simulink model "hil_demo"  (R2020a)
settings: Solver=VariableStepAuto  StartTime=0.0  StopTime=30  RelTol=1e-3
undefined symbols (not defined in the file): frame, physconst, system, UE
libraries: commsync2 x3, commsink2 x2, commdigbbndpm3 x2, commfilt2 x2, commsequence2 x2, phasedbflib x2, dspmathops x1, phaseddoalib x1, commrfcorlib x1, commutil2 x1, dspstat3 x1, dspsrcs4 x1
settings Model: Creator=jose_  LastModifiedBy=jose_

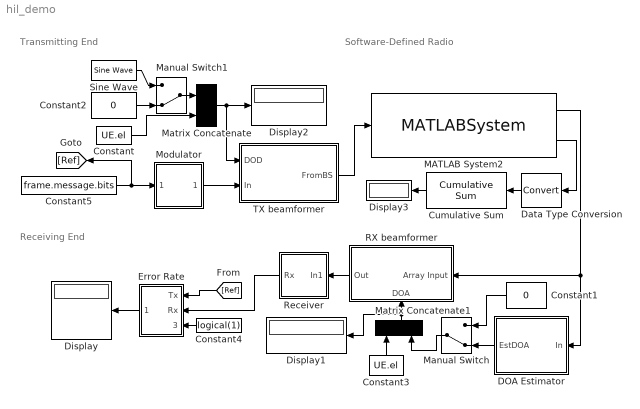
== system hil_demo ==
  note: Receiving End
  note: Software-Defined Radio
  note: Transmitting End
  Constant : Constant  Value=UE.el
  Constant1 : Constant  Value=0
  Constant2 : Constant  Value=0
  Constant3 : Constant  Value=UE.el
  Constant4 : Constant  Value=logical(1)
  Constant5 : Constant  Value=frame.message.bits  SampleTime=system.step
  Cumulative Sum : dspmathops/Cumulative Sum  dim=Channels (running sum)  reset_popup=None  roundingMode=Floor  overflowMode=off  outputDataTypeStr=Inherit: Same as accumulator  outputMin=[]  outputMax=[]  outputLastDataTypeStr=Inherit: Same as accumulator
  DOA Estimator : Subsystem
      mask Display: image('$imagefile'); % Use "Edit Image" on toolstrip to change.
  Data Type Conversion : DataTypeConversion
  Display{,1..3} (4 alike) : Display
  Error Rate : Subsystem
  MATLAB System2 : MATLABSystem  System=bladeRF_MIMO_Simulink  loopback_mode=None  xb200=off  SimulateUsing=Interpreted execution  enable_rx=on  enable_overrun=on  rx_frequency=system.freq  rx_samplerate=SDR.samplerate  rx_bandwidth=1.5  rx_gain=SDR.rx_gain  enable_rx_biastee=off  rx_agc=MANUAL  rx_num_buffers=SDR.stream.n_buffers  rx_num_transfers=SDR.stream.n_transfers  rx_buf_size=SDR.stream.buffer_size  rx_timeout_ms=SDR.stream.timeout  rx_step_size=SDR.samples_per_step  enable_tx=on  enable_underrun=off  tx_frequency=system.freq  tx_samplerate=SDR.samplerate  tx_bandwidth=1.5  tx_gain=SDR.tx_gain  enable_tx_biastee=off  tx_num_buffers=SDR.stream.n_buffers  tx_num_transfers=SDR.stream.n_transfers  tx_buf_size=SDR.stream.buffer_size  tx_timeout_ms=SDR.stream.timeout  tx_step_size=SDR.samples_per_step  verbosity=Verbose
      mask Type: bladeRF_MIMO_Simulink
      mask Display:
      | disp(['Nuand' char(10) 'bladeRF 2.0' char(10) 'MIMO']);
      | port_label('input',1,'TX Samples');
      | port_label('output',1,'RX Samples');
      | port_label('output',2,'RX Overrun');
  Manual Switch : ManualSwitch  CurrentSetting=0
  Manual Switch1 : ManualSwitch  CurrentSetting=0
  Matrix Concatenate : Concatenate  Mode=Multidimensional array
  Matrix Concatenate1 : Concatenate  Mode=Multidimensional array
  Modulator : Subsystem
      mask Display: image('$imagefile'); % Use "Edit Image" on toolstrip to change.
  RX beamformer : Subsystem
      settings: PortSchema="{\"entries\":[{\"content\":{\"sides\":[{\"content\":{\"connectorIds\":[\"In1\"]},\"type\":\"ConnectorPlacement.EquallySpacedRectSide\",\"uuid\":\"da6b99b9-07c1-40ec-94f6-5f8421c86696\"},{\"content\":{\"connectorIds\":[\"Out1\"],\"side\":\"RIGHT\"},\"type\":\"ConnectorPlacement.EquallySpacedRectSide\",\"uuid\":\"d1696111-4bb2-4715-9875-a9a0a5fdf0a8\"},{\"content\":{\"connectorIds\":[],\"side\":\"TOP\"},\"type\":\"ConnectorPlacement.EquallySpacedRectSide\",\"uuid\":\"2098a05d-1eb1-4caf-b28b-c43268db6279\"},{\"content\":{\"connectorIds\":[\"In2\"],\"side\":\"BOTTOM\"},\"type\":\"ConnectorPlacement.EquallySpacedRectSide\",\"uuid\":\"baaf1a26-1617-49ff-8044-4db1bbf8bae7\"}]},\"type\":\"ConnectorPlacement.EquallySpacedConnector\",\"uuid\":\"7953a551-d915-4cd7-8910-f2df4fb3e1ef\"}],\"packageUris\":[\"http://schema.mathworks.com/mf0/Connector/19700101\"],\"version\":\"1.0\"}"
      mask Display: image('$imagefile'); % Use "Edit Image" on toolstrip to change.
  Receiver : Subsystem
      mask Display: image('$imagefile'); % Use "Edit Image" on toolstrip to change.
  Sine Wave : dspsrcs4/Sine Wave  Amplitude=30  Frequency=0.1  Phase=0  SampleMode=Discrete  OutComplex=Real  CompMethod=Table lookup  TableSize=Speed  SampleTime=system.step  SamplesPerFrame=1  ResetState=Restart at time zero  OutputFrames=off  dataType=double  wordLen=16  udDataType=sfix(16)  fracBitsMode=Best precision  numFracBits=15  OutDataTypeStr=double  LastOutDataTypeStr=double
  TX beamformer : Subsystem
      mask Display: image('$imagefile'); % Use "Edit Image" on toolstrip to change.
  wires:
  Constant5/1 -> [Ref], Modulator/1(Message)
  TX beamformer/1(FromBS) -> MATLAB System2/1
  MATLAB System2/2 -> Data Type Conversion/1
  Data Type Conversion/1 -> Cumulative Sum/1
  Cumulative Sum/1 -> Display3/1
  RX beamformer/1(Out) -> Receiver/1(In1)
  Receiver/1(Rx) -> Error Rate/2(Rx)
  Error Rate/1(BER) -> Display/1
  [Ref] -> Error Rate/1(Tx)
  Constant4/1 -> Error Rate/3(Rst)
  MATLAB System2/1 -> RX beamformer/1(Array Input), DOA Estimator/1(In)
  DOA Estimator/1(EstDOA) -> Manual Switch/2
  Constant1/1 -> Manual Switch/1
  Modulator/1(Out1) -> TX beamformer/2(In)
  Constant2/1 -> Manual Switch1/2
  Matrix Concatenate/1 -> Display2/1, TX beamformer/1(DOD)
  Sine Wave/1 -> Manual Switch1/1
  Constant/1 -> Matrix Concatenate/2
  Manual Switch1/1 -> Matrix Concatenate/1
  Matrix Concatenate1/1 -> Display1/1, RX beamformer/2(DOA)
  Manual Switch/1 -> Matrix Concatenate1/2
  Constant3/1 -> Matrix Concatenate1/1

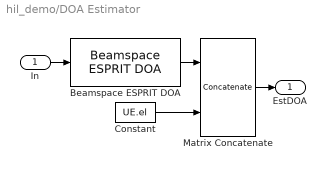
== system hil_demo/DOA Estimator ==
  In : Inport
  Beamspace ESPRIT DOA : phaseddoalib/Beamspace ESPRIT DOA  PropagationSpeed=physconst( 'LightSpeed' )  OperatingFrequency=system.freq  NumSignalsSource=Property  NumSignalsMethod=AIC  NumSignals=1  SpatialSmoothing=0  Method=TLS  BeamFanCenter=0  NumBeamsSource=Auto  NumBeams=1  SimulateUsing=Code generation  SensorArray=AntennaArray
      settings: SourceProductBaseCode=AR
  Constant : Constant  Value=UE.el
  Matrix Concatenate : Concatenate  Mode=Multidimensional array
  EstDOA : Outport
  wires:
  In/1 -> Beamspace ESPRIT DOA/1
  Beamspace ESPRIT DOA/1 -> Matrix Concatenate/1
  Matrix Concatenate/1 -> EstDOA/1
  Constant/1 -> Matrix Concatenate/2

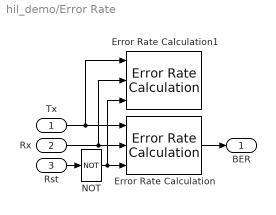
== system hil_demo/Error Rate ==
  Tx : Inport
  Rx : Inport  Port=2
  Rst : Inport  Port=3
  Error Rate Calculation : commsink2/Error Rate Calculation  N=0  st_delay=0  cp_mode=Entire frame  subframe=[]  PMode=Port  WsName=ErrorVec  RsMode2=on  stop=off  numErr=100  maxBits=1e6
  Error Rate Calculation1 : commsink2/Error Rate Calculation  N=0  st_delay=0  cp_mode=Entire frame  subframe=[]  PMode=Workspace  WsName=ErrorVec  RsMode2=on  stop=off  numErr=100  maxBits=1e6
  NOT : Logic  Operator=NOT  IconShape=distinctive  AllPortsSameDT=off  OutDataTypeStr=boolean
  BER : Outport
  wires:
  Tx/1 -> Error Rate Calculation1/1, Error Rate Calculation/1
  Rx/1 -> Error Rate Calculation1/2, Error Rate Calculation/2
  Error Rate Calculation/1 -> BER/1
  Rst/1 -> NOT/1
  NOT/1 -> Error Rate Calculation1/3, Error Rate Calculation/3

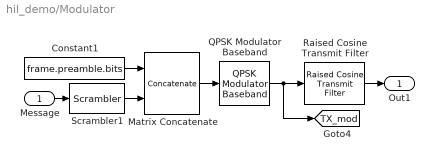
== system hil_demo/Modulator ==
  Message : Inport
  Constant1 : Constant  Value=frame.preamble.bits  SampleTime=system.step
  Matrix Concatenate : Concatenate  Mode=Multidimensional array
  QPSK Modulator Baseband : commdigbbndpm3/QPSK Modulator Baseband  InType=Bit  Enc=Gray  Ph=system.mod.PhaseOffset  outDtype=double  outWordLen=16  outUDDataType=sfix(16)  outFracLenMode=Best precision  outFracLen=15  outDataTypeStr=double  outLastDataTypeStr=double
  Raised Cosine Transmit Filter : commfilt2/Raised Cosine Transmit Filter  filtType=Square root  R=system.tx.rc.rolloff  filtSpan=system.tx.rc.span  N=system.tx.rc.interpolation  filterGain=1  InputProcessing=Columns as channels (frame based)  RateOptions=Enforce single-rate processing  framing=Mute  checkCoeff=off  variableName=rcTxFilt  checkGain=Normalized  sampMode=Mute  saveAsFlag=0  currentFiltSpan=system.tx.rc.span  D=(system.tx.rc.span)/2  launchFVT=on  roundingMode=Floor  overflowMode=off  coeffDataTypeStr=Inherit: Same word length as input  coeffMin=[]  coeffMax=[]  coeffLastDataTypeStr=Inherit: Same word length as input  outputDataTypeStr=Inherit: Same as accumulator  outputMin=[]  outputMax=[]  outputLastDataTypeStr=Inherit: Same as accumulator
  Scrambler1 : commsequence2/Scrambler  M=2  poly=[1 1 1 0 1]  iniStaSource=Dialog Parameter  ini_sta=[0 0 0 0]  resetViaPort=off
      settings: SourceProductBaseCode=CM
  Out1 : Outport
  tag scope: TX_mod=global
  wires:
  QPSK Modulator Baseband/1 -> [TX_mod], Raised Cosine Transmit Filter/1
  Matrix Concatenate/1 -> QPSK Modulator Baseband/1
  Raised Cosine Transmit Filter/1 -> Out1/1
  Constant1/1 -> Matrix Concatenate/1
  Message/1 -> Scrambler1/1
  Scrambler1/1 -> Matrix Concatenate/2

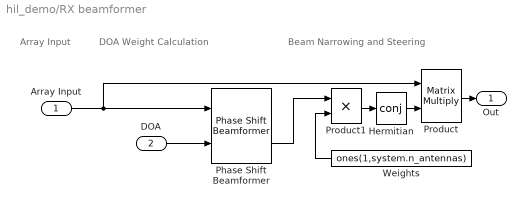
== system hil_demo/RX beamformer ==
  note: Beam Narrowing and Steering
  note: DOA Weight Calculation
  note: Array Input
  Array Input : Inport
  DOA : Inport  Port=2
  Hermitian : Math  Operator=conj  SaturateOnIntegerOverflow=on
  Phase Shift Beamformer : phasedbflib/Phase Shift Beamformer  PropagationSpeed=physconst( 'LightSpeed' )  OperatingFrequency=system.freq  DirectionSource=Input port  Direction=[ 0; 0 ]  NumPhaseShifterBits=0  WeightsNormalization=Preserve power  WeightsOutputPort=on  SimulateUsing=Code generation  SensorArray=AntennaArray
      settings: SourceProductBaseCode=AR
  Product : Product  Multiplication=Matrix(*)
  Product1 : Product
  Weights : Constant  Value=ones(1,system.n_antennas)
  Out : Outport
  wires:
  Product1/1 -> Hermitian/1
  Hermitian/1 -> Product/2
  Product/1 -> Out/1
  Weights/1 -> Product1/2
  Phase Shift Beamformer/2 -> Product1/1
  Array Input/1 -> Product/1, Phase Shift Beamformer/1
  DOA/1 -> Phase Shift Beamformer/2

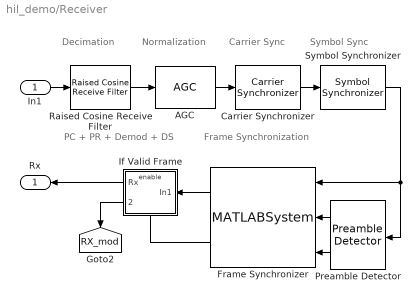
== system hil_demo/Receiver ==
  note: PC + PR + Demod + DS
  note: Frame Synchronization
  note: Symbol Sync
  note: Carrier Sync
  note: Normalization
  note: Decimation
  In1 : Inport
  AGC : commrfcorlib/AGC  LegacyMode=off  DetectorMethod=Rectifier  LoopMethod=Linear  UpdatePeriod=100  StepSize=0.1  AdaptationStepSize=system.rx.agc.step  DesiredOutputPower=system.rx.agc.output_power  AveragingLength=system.rx.agc.average_length  MaximumGain=30  MaxPowerGain=system.rx.agc.max_power  GainOutputPort=off  InputPowerOutputPort=off  SimulateUsing=Code generation
  Carrier Synchronizer : commsync2/Carrier Synchronizer  Modulation=QPSK  ModulationPhaseOffset=Auto  CustomPhaseOffset=0  SamplesPerSymbol=system.rx.cs.sps  DampingFactor=system.rx.cs.damp  NormalizedLoopBandwidth=system.rx.cs.bandwidth  EstimatedPhaseErrorOutputPort=off  SimulateUsing=Code generation
  Frame Synchronizer : MATLABSystem  System=comm.internal.examples.FrameSynchronizer  Input=Symbol  OutputFrameLength=system.rx.fs.frame_length  PreambleLength=system.rx.fs.preamble_length  SimulateUsing=Code generation
      mask Type: comm.internal.examples.FrameSynchronizer
      mask Display:
      | disp(['Frame' char(10) 'Synchronizer']);
      | port_label('input',1,'u');
      | port_label('input',2,'idx');
      | port_label('input',3,'dtMt');
      | port_label('output',1,'Frame');
      | port_label('output',2,'Valid');
  If Valid Frame : Subsystem  TreatAsAtomicUnit=on
  Preamble Detector : commsync2/Preamble Detector  Input=Symbol  Preamble=system.rx.pd.preamble  Threshold=system.rx.pd.threshold  DetectionMetricOutput=on  Detections=All  SimulateUsing=Code generation
      settings: SourceProductBaseCode=CM
  Raised Cosine Receive Filter : commfilt2/Raised Cosine Receive Filter  filtType=Square root  R=system.rx.rc.rolloff  filtSpan=system.rx.rc.span  N=system.rx.rc.sps  downFactor=system.rx.rc.decimation  downOffset=0  filterGain=1  InputProcessing=Columns as channels (frame based)  RateOptions=Enforce single-rate processing  framing=Mute  checkCoeff=off  variableName=rcRxFilt  currentFiltSpan=system.rx.rc.span  D=(system.rx.rc.span)/2  inputOffset=0  sampMode=Mute  saveAsFlag=0  rateMode=Downsampling  checkGain=Normalized  launchFVT=on  roundingMode=Floor  overflowMode=off  coeffDataTypeStr=Inherit: Same word length as input  coeffMin=[]  coeffMax=[]  coeffLastDataTypeStr=Inherit: Same word length as input  accumDataTypeStr=Inherit: Same as product output  accumLastDataTypeStr=Inherit: Same as product output  outputDataTypeStr=Inherit: Same as accumulator  outputMin=[]  outputMax=[]  outputLastDataTypeStr=Inherit: Same as accumulator
  Symbol Synchronizer : commsync2/Symbol Synchronizer  Modulation=PAM/PSK/QAM  TimingErrorDetector=Zero-Crossing (decision-directed)  SamplesPerSymbol=system.rx.ss.sps  DampingFactor=system.rx.ss.damp  NormalizedLoopBandwidth=system.rx.ss.bandwidth  DetectorGain=system.rx.ss.gain  TimingErrorOutputPort=off  SimulateUsing=Code generation
      settings: SourceProductBaseCode=CM
  Rx : Outport
  tag scope: RX_mod=global
  wires:
  In1/1 -> Raised Cosine Receive Filter/1
  Raised Cosine Receive Filter/1 -> AGC/1
  Preamble Detector/1 -> Frame Synchronizer/2
  Frame Synchronizer/1 -> If Valid Frame/1(In1)
  If Valid Frame/1(Rx) -> Rx/1
  Frame Synchronizer/2 -> If Valid Frame/Enable
  AGC/1 -> Carrier Synchronizer/1
  Carrier Synchronizer/1 -> Symbol Synchronizer/1
  Preamble Detector/2 -> Frame Synchronizer/3
  Symbol Synchronizer/1 -> Frame Synchronizer/1, Preamble Detector/1
  If Valid Frame/2(pre-demod) -> [RX_mod]

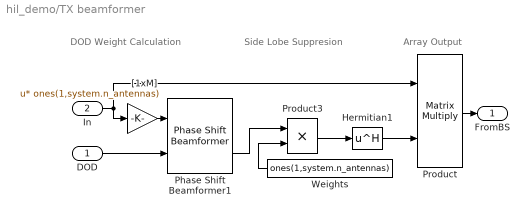
== system hil_demo/TX beamformer ==
  note: Array Output
  note: Side Lobe Suppresion
  note: DOD Weight Calculation
  DOD : Inport
  In : Inport  Port=2
  Hermitian1 : Math  Operator=hermitian  SaturateOnIntegerOverflow=on
  Phase Shift Beamformer1 : phasedbflib/Phase Shift Beamformer  PropagationSpeed=physconst( 'LightSpeed' )  OperatingFrequency=system.freq  DirectionSource=Input port  Direction=[ 0; 0 ]  NumPhaseShifterBits=0  WeightsNormalization=Preserve power  WeightsOutputPort=on  SimulateUsing=Code generation  SensorArray=AntennaArray
      settings: SourceProductBaseCode=AR
  Product : Product  Multiplication=Matrix(*)
  Product3 : Product
  Weights : Constant  Value=ones(1,system.n_antennas)  SampleTime=system.step
  "[1xM]" : Gain  Gain=ones(1,system.n_antennas)  Multiplication=Matrix(u*K)
  FromBS : Outport
  wires:
  Weights/1 -> Product3/2
  Phase Shift Beamformer1/2 -> Product3/1
  DOD/1 -> Phase Shift Beamformer1/2
  Hermitian1/1 -> Product/2
  Product3/1 -> Hermitian1/1
  Product/1 -> FromBS/1
  In/1 -> "[1xM]"/1, Product/1
  "[1xM]"/1 -> Phase Shift Beamformer1/1

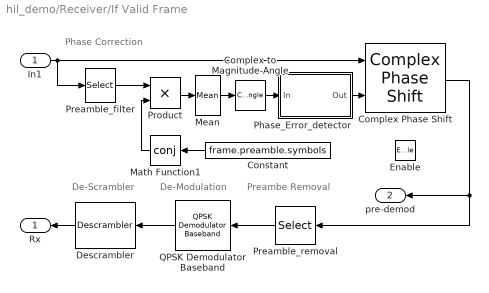
== system hil_demo/Receiver/If Valid Frame ==
  note: De-Scrambler
  note: De-Modulation
  note: Preambe Removal
  note: Phase Correction
  In1 : Inport
  Enable : EnablePort
  Complex Phase Shift : commutil2/Complex Phase Shift
      settings: SourceProductBaseCode=CM
  Complex to Magnitude-Angle : ComplexToMagnitudeAngle  Output=Angle
  Constant : Constant  Value=frame.preamble.symbols
  Descrambler : commsequence2/Descrambler  M=2  poly=[1 1 1 0 1]  iniStaSource=Dialog Parameter  ini_sta=[0 0 0 0]  resetViaPort=off
      settings: SourceProductBaseCode=CM
  Math Function1 : Math  Operator=conj  SignedPower=on  SaturateOnIntegerOverflow=on
  Mean : dspstat3/Mean  run=off  InputProcessing=Columns as channels (frame based)  reset_popup=None  directionMode=Each column  dimension=1  roiEnable=off  roiType=Rectangles  roiPortion=Entire ROI  roiOutput=Individual statistics for each ROI  roiFlag=off  roundingMode=Floor  overflowMode=off  outputDataTypeStr=Inherit: Same as accumulator  outputMin=[]  outputMax=[]  outputLastDataTypeStr=Inherit: Same as accumulator
  Phase_Error_detector : MATLAB Function  TreatAsAtomicUnit=on
  Preamble_filter : Selector  InputPortWidth=length(frame.symbols)  IndexOptions=Index vector (dialog)  Indices=1:length(frame.preamble.symbols)  OutputSizes=1
  Preamble_removal : Selector  InputPortWidth=length(frame.symbols)  IndexOptions=Index vector (dialog)  Indices=(length(frame.preamble.symbols)+1):length(frame.symbols)  OutputSizes=1
  Product : Product  RndMeth=Zero
  QPSK Demodulator Baseband : commdigbbndpm3/QPSK Demodulator Baseband  OutType=Bit  DecType=Hard decision  VarSource=Dialog  Variance=1  Dec=Gray  Ph=system.mod.PhaseOffset  outDtype1=Inherit via internal rule  outDtype2=Inherit via internal rule  derotateFactorWordLen=16  derotateFactorDataTypeStr=Inherit: Same word length as input  derotateFactorLastDataTypeStr=Inherit: Same word length as input
  Rx : Outport
  pre-demod : Outport  Port=2
  wires:
  Mean/1 -> Complex to Magnitude-Angle/1
  Product/1 -> Mean/1
  Complex to Magnitude-Angle/1 -> Phase_Error_detector/1(In)
  Preamble_filter/1 -> Product/1
  In1/1 -> Preamble_filter/1, Complex Phase Shift/1
  Constant/1 -> Math Function1/1
  Phase_Error_detector/1(Out) -> Complex Phase Shift/2
  Complex Phase Shift/1 -> Preamble_removal/1, pre-demod/1
  Math Function1/1 -> Product/2
  Preamble_removal/1 -> QPSK Demodulator Baseband/1
  QPSK Demodulator Baseband/1 -> Descrambler/1
  Descrambler/1 -> Rx/1

== matlab function hil_demo/Receiver/If Valid Frame/Phase_Error_detector ==
  data: In input; Out output
function Out = phasedecision(In)
% Map the estimated phase to one of -pi, -pi/2, 0, pi/2,  
%#codegen
Out = -round(In.*2./pi)./2.*pi;
% The above processing is equivalent to the following processing using
% if/else statements
%
% if In<pi/4 && In>-pi/4
%     Out = 0;
% elseif In>=pi/4 && In<pi*3/4
%     Out = pi/2;
% elseif In>=pi*3/4 || In<=-pi*3/4
%     Out = -pi;
% else
%     Out = -pi/2;
% end
